simulink model "EvPowertrainController4EM"  (R2024b)
settings: configuration reference "VehicleFixed10ms" (kept outside this file)
model workspace (MAT data in the model file):
  CtrlVcuAccelPdlBpts = [0 0.8 1]
  CtrlVcuBattPnlty = 10000000
  CtrlVcuBattSOCBpts = [0 20 60 80 100]
  CtrlVcuCnstrntPnltyFctr = 10000000
  CtrlVcuEMPnlty = 100
  CtrlVcuEMTrqSplitGrid = 200
  CtrlVcuFallRate = -500
  CtrlVcuMaxAccelG = 1
  CtrlVcuMaxDecelG = -1.5
  CtrlVcuPwrDeltaPnlty = 50
  CtrlVcuPwrRatePnlty = [25 25 100]
  CtrlVcuRiseRate = 500
  CtrlVcuRoadMuEst = 0.8
  CtrlVcuSftyFctr = 0.9
  CtrlVcuTracPwrErrPnlty = 25
  CtrlVcuTrqVecBrkThresh = 0.01
  CtrlVcuTrqVecIGain = 0
  CtrlVcuTrqVecMinTrq = 25
  CtrlVcuTrqVecPGain = -2000
  CtrlVcuTrqVecSteerThresh = 0.349065850399
  CtrlVcuTrqVecVelThresh = 2.5
  N_P0 = 3
undefined symbols (not defined in the file): CtrlBcuTrlrBrkGain, CtrlVcuEvChrgLmtBpt, CtrlVcuEvRegenBrkCutOff, CtrlVcuEvRegenBrkSpdBpt, CtrlVcuEvSocBpt, eff, EnvGrvty, PlntBrkActrBoreFrnt, PlntBrkFrntBias, PlntBrkKinFricCffFrnt, PlntBrkNumPadsFrnt, PlntBrkPadMeanRadiusFrnt, PlntBrkPrsFctr, PlntBrkRearBias, PlntDiffrntl2Eff, PlntDiffrntl2Ratio, PlntDiffrntlEff, PlntDiffrntlRatio, PlntEM1EffTbl, PlntEM1Spd, PlntEM1SpdEff, PlntEM1Trq, PlntEM1TrqEff, PlntEM2EffTbl, PlntEM2Spd, PlntEM2SpdEff, PlntEM2Trq, PlntEM2TrqEff, PlntEM3EffTbl, PlntEM3Spd, PlntEM3SpdEff, PlntEM3Trq, PlntEM3TrqEff, PlntEMWhlGearEffFL, PlntEMWhlGearEffRL, PlntEMWhlGearRatioFL, PlntEMWhlGearRatioRL, PlntTransEffSpdBpt, PlntTransEffTbl, PlntTransEffTempBpt, PlntTransEffTrqBpt, PlntTransGearNumVect, PlntTransGearRatioVect, PlntVehCGHgtAxl, PlntVehDstCGFrntAxl, PlntVehDstCGRearAxl, PlntVehMass, PlntWhlLdRadiusFrnt, PlntWhlLdRadiusRear
libraries: simulink x25, autolibutils x2, slpidlib x2
(part 6 of 7)

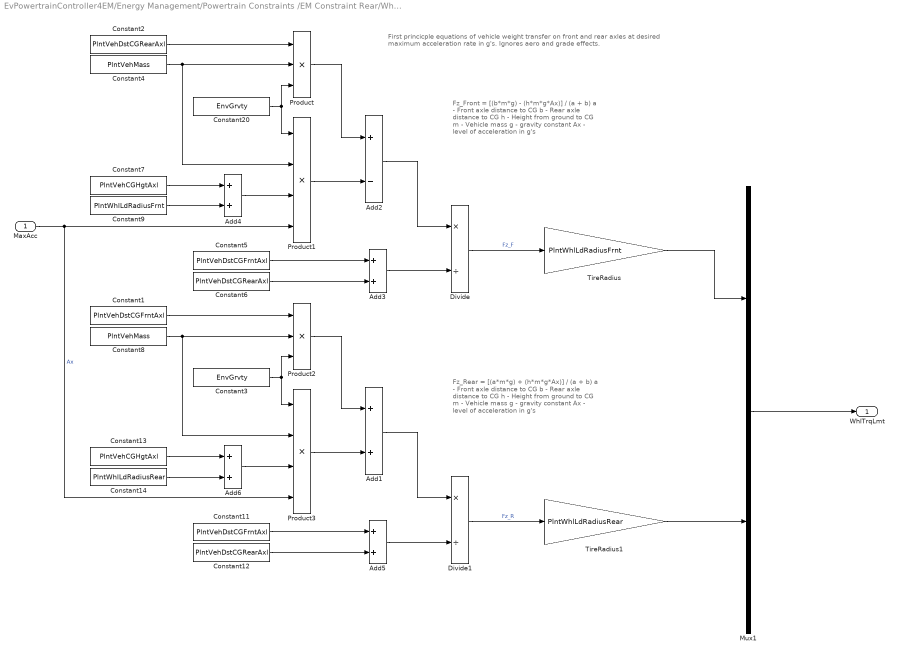
== system EvPowertrainController4EM/Energy Management/Powertrain Constraints /EM Constraint Rear/Wheel Torque Saturation for Max g Rates/Wheel Torque Limit at Max g Rates/Wheel Torque at Max Acceleration Rate ==
  note: Fz_Rear = [(a*m*g) + (h*m*g*Ax)] / (a + b)
      |
      | a - Front axle distance to CG
      | b - Rear axle distance to CG
      | h - Height from ground to CG
      | m - Vehicle mass
      | g - gravity constant
      | Ax - level of acceleration in g's
  note: Fz_Front = [(b*m*g) - (h*m*g*Ax)] / (a + b)
      |
      | a - Front axle distance to CG
      | b - Rear axle distance to CG
      | h - Height from ground to CG
      | m - Vehicle mass
      | g - gravity constant
      | Ax - level of acceleration in g's
  note: First princicple equations of vehicle weight transfer on front
      | and rear axles at desired maximum acceleration rate in g's.
      | Ignores aero and grade effects.
  MaxAcc : Inport
  Add{1,3..6} (5 alike) : Sum
  Add2 : Sum  Inputs=+-
  Constant1 : Constant  Value=PlntVehDstCGFrntAxl  SampleTime=-1
  Constant11 : Constant  Value=PlntVehDstCGFrntAxl  SampleTime=-1
  Constant12 : Constant  Value=PlntVehDstCGRearAxl  SampleTime=-1
  Constant13 : Constant  Value=PlntVehCGHgtAxl  SampleTime=-1
  Constant14 : Constant  Value=PlntWhlLdRadiusRear  SampleTime=-1
  Constant2 : Constant  Value=PlntVehDstCGRearAxl  SampleTime=-1
  Constant20 : Constant  Value=EnvGrvty  SampleTime=-1
  Constant3 : Constant  Value=EnvGrvty  SampleTime=-1
  Constant4 : Constant  Value=PlntVehMass  SampleTime=-1
  Constant5 : Constant  Value=PlntVehDstCGFrntAxl  SampleTime=-1
  Constant6 : Constant  Value=PlntVehDstCGRearAxl  SampleTime=-1
  Constant7 : Constant  Value=PlntVehCGHgtAxl  SampleTime=-1
  Constant8 : Constant  Value=PlntVehMass  SampleTime=-1
  Constant9 : Constant  Value=PlntWhlLdRadiusFrnt  SampleTime=-1
  Divide : Product  Inputs=*/
  Divide1 : Product  Inputs=*/
  Mux1 : Mux  Inputs=2
  Product : Product  Inputs=3
  Product1 : Product  Inputs=4
  Product2 : Product  Inputs=3
  Product3 : Product  Inputs=4
  TireRadius : Gain  Gain=PlntWhlLdRadiusFrnt
  TireRadius1 : Gain  Gain=PlntWhlLdRadiusRear
  WhlTrqLmt : Outport  VectorParamsAs1DForOutWhenUnconnected=off
  wires:
  Divide1/1 -> TireRadius1/1  "Fz_R"
  Product3/1 -> Add1/2
  Product2/1 -> Add1/1
  Constant11/1 -> Add5/1
  Constant8/1 -> Product3/2, Product2/2
  Add5/1 -> Divide1/2
  Add6/1 -> Product3/3
  Constant12/1 -> Add5/2
  Constant1/1 -> Product2/1
  Constant13/1 -> Add6/1
  Constant14/1 -> Add6/2
  Add1/1 -> Divide1/1
  Constant3/1 -> Product3/1, Product2/3
  Constant20/1 -> Product/3, Product1/1
  Mux1/1 -> WhlTrqLmt/1
  Add2/1 -> Divide/1
  Constant9/1 -> Add4/2
  Constant7/1 -> Add4/1
  Constant2/1 -> Product/1
  Constant6/1 -> Add3/2
  Divide/1 -> TireRadius/1  "Fz_F"
  Add4/1 -> Product1/3
  Add3/1 -> Divide/2
  MaxAcc/1 -> Product1/4, Product3/4  "Ax"
  Constant4/1 -> Product/2, Product1/2
  Constant5/1 -> Add3/1
  Product/1 -> Add2/1
  Product1/1 -> Add2/2
  TireRadius/1 -> Mux1/1
  TireRadius1/1 -> Mux1/2

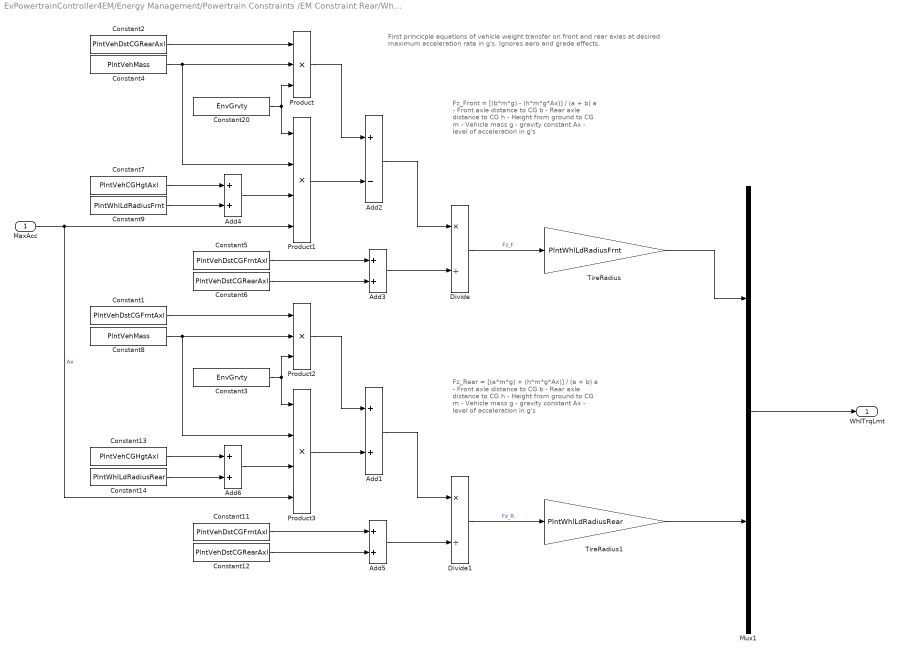
== system EvPowertrainController4EM/Energy Management/Powertrain Constraints /EM Constraint Rear/Wheel Torque Saturation for Max g Rates/Wheel Torque Limit at Max g Rates/Wheel Torque at Max Deceleration Rate ==
  note: First princicple equations of vehicle weight transfer on front
      | and rear axles at desired maximum acceleration rate in g's.
      | Ignores aero and grade effects.
  note: Fz_Front = [(b*m*g) - (h*m*g*Ax)] / (a + b)
      |
      | a - Front axle distance to CG
      | b - Rear axle distance to CG
      | h - Height from ground to CG
      | m - Vehicle mass
      | g - gravity constant
      | Ax - level of acceleration in g's
  note: Fz_Rear = [(a*m*g) + (h*m*g*Ax)] / (a + b)
      |
      | a - Front axle distance to CG
      | b - Rear axle distance to CG
      | h - Height from ground to CG
      | m - Vehicle mass
      | g - gravity constant
      | Ax - level of acceleration in g's
  MaxAcc : Inport
  Add{1,3..6} (5 alike) : Sum
  Add2 : Sum  Inputs=+-
  Constant1 : Constant  Value=PlntVehDstCGFrntAxl  SampleTime=-1
  Constant11 : Constant  Value=PlntVehDstCGFrntAxl  SampleTime=-1
  Constant12 : Constant  Value=PlntVehDstCGRearAxl  SampleTime=-1
  Constant13 : Constant  Value=PlntVehCGHgtAxl  SampleTime=-1
  Constant14 : Constant  Value=PlntWhlLdRadiusRear  SampleTime=-1
  Constant2 : Constant  Value=PlntVehDstCGRearAxl  SampleTime=-1
  Constant20 : Constant  Value=EnvGrvty  SampleTime=-1
  Constant3 : Constant  Value=EnvGrvty  SampleTime=-1
  Constant4 : Constant  Value=PlntVehMass  SampleTime=-1
  Constant5 : Constant  Value=PlntVehDstCGFrntAxl  SampleTime=-1
  Constant6 : Constant  Value=PlntVehDstCGRearAxl  SampleTime=-1
  Constant7 : Constant  Value=PlntVehCGHgtAxl  SampleTime=-1
  Constant8 : Constant  Value=PlntVehMass  SampleTime=-1
  Constant9 : Constant  Value=PlntWhlLdRadiusFrnt  SampleTime=-1
  Divide : Product  Inputs=*/
  Divide1 : Product  Inputs=*/
  Mux1 : Mux  Inputs=2
  Product : Product  Inputs=3
  Product1 : Product  Inputs=4
  Product2 : Product  Inputs=3
  Product3 : Product  Inputs=4
  TireRadius : Gain  Gain=PlntWhlLdRadiusFrnt
  TireRadius1 : Gain  Gain=PlntWhlLdRadiusRear
  WhlTrqLmt : Outport  VectorParamsAs1DForOutWhenUnconnected=off
  wires:
  TireRadius1/1 -> Mux1/2
  TireRadius/1 -> Mux1/1
  Product1/1 -> Add2/2
  Product/1 -> Add2/1
  Constant5/1 -> Add3/1
  Constant4/1 -> Product1/2, Product/2
  MaxAcc/1 -> Product3/4, Product1/4  "Ax"
  Add3/1 -> Divide/2
  Add4/1 -> Product1/3
  Divide/1 -> TireRadius/1  "Fz_F"
  Constant6/1 -> Add3/2
  Constant2/1 -> Product/1
  Constant7/1 -> Add4/1
  Constant9/1 -> Add4/2
  Add2/1 -> Divide/1
  Mux1/1 -> WhlTrqLmt/1
  Constant20/1 -> Product1/1, Product/3
  Constant3/1 -> Product2/3, Product3/1
  Add1/1 -> Divide1/1
  Constant14/1 -> Add6/2
  Constant13/1 -> Add6/1
  Constant1/1 -> Product2/1
  Constant12/1 -> Add5/2
  Add6/1 -> Product3/3
  Add5/1 -> Divide1/2
  Constant8/1 -> Product2/2, Product3/2
  Constant11/1 -> Add5/1
  Product2/1 -> Add1/1
  Product3/1 -> Add1/2
  Divide1/1 -> TireRadius1/1  "Fz_R"

== system EvPowertrainController4EM/Energy Management/Powertrain Constraints /EM Constraint Front/Tabular Power Loss Data/2EM or 3EM Dual Rear/WhlTrq2EMTrq/Diff Eta ==
  note: Pwr >= 0, v = 1
      | Pwr < 0, v= -1
  SpdIn : Inport
  TrqIn : Inport  Port=2
  Constant : Constant  Value=PlntDiffrntl2Eff
  Constant1 : Constant  SampleTime=-1
  Constant2 : Constant  Value=-1  SampleTime=-1
  Math Function1 : Math  Operator=pow  SignedPower=on  OutputSignalType=real
  Product1 : Product
  Switch2 : Switch  SaturateOnIntegerOverflow=off  InputSameDT=off
  eta : Outport  VectorParamsAs1DForOutWhenUnconnected=off
  wires:
  SpdIn/1 -> Product1/2
  Constant/1 -> Math Function1/1
  Constant2/1 -> Switch2/3
  Constant1/1 -> Switch2/1
  Product1/1 -> Switch2/2
  Switch2/1 -> Math Function1/2
  Math Function1/1 -> eta/1
  TrqIn/1 -> Product1/1

== system EvPowertrainController4EM/Energy Management/Powertrain Constraints /EM Constraint Front/Tabular Power Loss Data/3EM Dual Front or 4EM/WhlTrq2EMTrq/Gear Eta ==
  note: Pwr >= 0, v = 1
      | Pwr < 0, v= -1
  SpdIn : Inport
  TrqIn : Inport  Port=2
  Constant : Constant  Value=PlntEMWhlGearEffRL
  Constant1 : Constant  SampleTime=-1
  Constant2 : Constant  Value=-1  SampleTime=-1
  Math Function1 : Math  Operator=pow  SignedPower=on  OutputSignalType=real
  Product1 : Product
  Switch2 : Switch  SaturateOnIntegerOverflow=off  InputSameDT=off
  eta : Outport  VectorParamsAs1DForOutWhenUnconnected=off
  wires:
  TrqIn/1 -> Product1/1
  Math Function1/1 -> eta/1
  Switch2/1 -> Math Function1/2
  Product1/1 -> Switch2/2
  Constant1/1 -> Switch2/1
  Constant2/1 -> Switch2/3
  Constant/1 -> Math Function1/1
  SpdIn/1 -> Product1/2

== system EvPowertrainController4EM/Energy Management/Powertrain Constraints /EM Constraint Rear/Tabular Power Loss Data/2EM/WhlTrq2EMTrq/Diff Eta ==
  note: Pwr >= 0, v = 1
      | Pwr < 0, v= -1
  SpdIn : Inport
  TrqIn : Inport  Port=2
  Constant : Constant  Value=PlntDiffrntl2Eff
  Constant1 : Constant  SampleTime=-1
  Constant2 : Constant  Value=-1  SampleTime=-1
  Math Function1 : Math  Operator=pow  SignedPower=on  OutputSignalType=real
  Product1 : Product
  Switch2 : Switch  SaturateOnIntegerOverflow=off  InputSameDT=off
  eta : Outport  VectorParamsAs1DForOutWhenUnconnected=off
  wires:
  SpdIn/1 -> Product1/2
  Constant/1 -> Math Function1/1
  Constant2/1 -> Switch2/3
  Constant1/1 -> Switch2/1
  Product1/1 -> Switch2/2
  Switch2/1 -> Math Function1/2
  Math Function1/1 -> eta/1
  TrqIn/1 -> Product1/1

== system EvPowertrainController4EM/Energy Management/Powertrain Constraints /EM Constraint Rear/Tabular Power Loss Data/3EM Dual Front/WhlTrq2EMTrq/Diff Eta ==
  note: Pwr >= 0, v = 1
      | Pwr < 0, v= -1
  SpdIn : Inport
  TrqIn : Inport  Port=2
  Constant : Constant  Value=PlntDiffrntl2Eff
  Constant1 : Constant  SampleTime=-1
  Constant2 : Constant  Value=-1  SampleTime=-1
  Math Function1 : Math  Operator=pow  SignedPower=on  OutputSignalType=real
  Product1 : Product
  Switch2 : Switch  SaturateOnIntegerOverflow=off  InputSameDT=off
  eta : Outport  VectorParamsAs1DForOutWhenUnconnected=off
  wires:
  TrqIn/1 -> Product1/1
  Math Function1/1 -> eta/1
  Switch2/1 -> Math Function1/2
  Product1/1 -> Switch2/2
  Constant1/1 -> Switch2/1
  Constant2/1 -> Switch2/3
  Constant/1 -> Math Function1/1
  SpdIn/1 -> Product1/2

== system EvPowertrainController4EM/Energy Management/Powertrain Constraints /EM Constraint Rear/Tabular Power Loss Data/3EM Dual Rear or 4EM/WhlTrq2EMTrq/Gear Eta ==
  note: Pwr >= 0, v = 1
      | Pwr < 0, v= -1
  SpdIn : Inport
  TrqIn : Inport  Port=2
  Constant : Constant  Value=PlntEMWhlGearEffRL
  Constant1 : Constant  SampleTime=-1
  Constant2 : Constant  Value=-1  SampleTime=-1
  Math Function1 : Math  Operator=pow  SignedPower=on  OutputSignalType=real
  Product1 : Product
  Switch2 : Switch  SaturateOnIntegerOverflow=off  InputSameDT=off
  eta : Outport  VectorParamsAs1DForOutWhenUnconnected=off
  wires:
  TrqIn/1 -> Product1/1
  Math Function1/1 -> eta/1
  Switch2/1 -> Math Function1/2
  Product1/1 -> Switch2/2
  Constant1/1 -> Switch2/1
  Constant2/1 -> Switch2/3
  Constant/1 -> Math Function1/1
  SpdIn/1 -> Product1/2

== matlab function EvPowertrainController4EM/Torque Vectoring/3EM/Torque Vectoring Split Function ==
  data: MaxTrq input; TrqLeftOut output; TrqLeft input; TrqRght input; TrqRghtOut output; TrqVec input; Enbl input; BrkThresh input; MinTrq input
function [TrqLeftOut, TrqRghtOut] = fcn(MaxTrq, TrqLeft, TrqRght, TrqVec, Enbl, BrkThresh, MinTrq)
% Enbl:= flag to turn on TV, true if steering wheel is turned and non-zero vehicle speed
% BrkThresh:= flag to turn on TV, true if not braking
TrqLmt = min(MaxTrq-abs(TrqLeft),MaxTrq-abs(TrqRght));
DeltaTrq = min(MinTrq, min(TrqLmt,abs(TrqVec)))*sign(TrqVec)*Enbl;% limit difference in torque between tires to +/-MinTrq and to max/min motor torque
if BrkThresh > 0 % Not braking. Use Torque vectoring
    TrqLeftOut = (TrqLeft+DeltaTrq);
    TrqRghtOut = (TrqRght-DeltaTrq);
else % ignore TV
    TrqLeftOut = TrqLeft;
    TrqRghtOut = TrqRght;
end

== matlab function EvPowertrainController4EM/Torque Vectoring/4EM/Torque Vectoring Split Function Rear ==
  data: MaxTrq input; TrqLeftOut output; TrqLeft input; TrqRght input; TrqRghtOut output; TrqVec input; Enbl input; BrkThresh input; MinTrq input
function [TrqLeftOut, TrqRghtOut] = fcn(MaxTrq, TrqLeft, TrqRght, TrqVec, Enbl, BrkThresh, MinTrq)
% Enbl:= flag to turn on TV, true if steering wheel is turned and non-zero vehicle speed
% BrkThresh:= flag to turn on TV, true if not braking
TrqLmt = min(MaxTrq-abs(TrqLeft),MaxTrq-abs(TrqRght));
DeltaTrq = min(MinTrq, min(TrqLmt,abs(TrqVec)))*sign(TrqVec)*Enbl;% limit difference in torque between tires to +/-MinTrq and to max/min motor torque
if BrkThresh > 0 % Not braking. Use Torque vectoring
    TrqLeftOut = (TrqLeft+DeltaTrq);
    TrqRghtOut = (TrqRght-DeltaTrq);
else % ignore TV
    TrqLeftOut = TrqLeft;
    TrqRghtOut = TrqRght;
end

== matlab function EvPowertrainController4EM/Torque Vectoring/LTV_MPC/LTV_MPCFcn ==
  data: Acc input; delta_Frnt input; TV_enableflag input; xk input; PrevEMTrqCmdFinals input; EMTrqCmds input; Vx input; EMTrqMaxFrnt input; EMTrqMaxRear input; xi_in input; EMTrqCmdFinal output; xhat_kp1 output; fval output; exitflag output; allCosts output; compTime output; stepSize output; iterations output; funcCount output; betaMax output; r_ref output; xi_out output
function [EMTrqCmdFinal, xhat_kp1, fval, exitflag, allCosts, compTime, stepSize, iterations, funcCount, betaMax, r_ref, xi_out] ...
    = LTV_MPC(Acc, delta_Frnt, TV_enableflag, xk, PrevEMTrqCmdFinals, EMTrqCmds, Vx, EMTrqMaxFrnt, EMTrqMaxRear, xi_in)

%% MPC Tuning Parameters
Np = 10;    % prediction horizon [interval]
Nc = 3;     % control horizon [interval] 

% % -----------------------------------------------------------------

Q_y = 100;      % Yaw rate tracking weight
Q_T = eye(4);  % Torque increment (slew rate) weight

% % -----------------------------------------------------------------

% % % Allowed Maximum MPC computation Iterations
Iter_max = 300;

%% Defining fixed parameter structure
nx = 2; % number of states
nu = 2; % number of controls

% % System parameters
m  = 1623;          % [kg]           % vehicle mass
Iz = 2066;          % [kg m^2]       % yaw moment of inertia
lf = 1.09;          % [m]            % distance from c.o.g. to front axle
lr = 1.7;           % [m]            % distance from c.o.g. to rear axle
lw = 1.575;         % [m]            % track width
rw = 0.309;         % [m]            % wheel radius
h  = 0.609;         % [m]            % distance from c.o.g. to ground
g  = 9.81;          % [m/s^2]        % gravitational acceleration

mu_x = 0.8*0.9;     % assumed tire-road friction coefficient

% % Tires' magic formula coefficients
D = 1.0;    % []            % peak factor scale
C = 1.1;    % []            % shape factor
E = 1.2;    % []            % curvature factor

EMWhlGearRatio = 0.98*4.1; % (wheel torque = efficiency * final gear * motor torque)

EMTrqIncMax = 500*0.01.*ones(4,1); % sampling time = 0.01 [s];

EMFrntTrq = EMTrqCmds(1) + EMTrqCmds(2); % front axle (motor) torque
EMRearTrq = EMTrqCmds(3) + EMTrqCmds(4); % rear  axle (motor) torque

%% System bounds
% % Maximum side slip angle
Car = 2.4E4; % (estimated) rear cornering stiffness
betaMax = abs(mu_x*g*(lr/Vx^2 + m*lf/(Car*(lf+lr))));

%% Yaw rate reference
% Neutral steer
r_ref = Vx*delta_Frnt/(lf+lr);

% Maximum yaw rate reference
r_ref_max = abs(0.85* mu_x*g/(Vx+1e-6)); 

% Saturated reference
if abs(r_ref) > r_ref_max
    r_ref = r_ref_max*sign(delta_Frnt);
end

%% Provide an initial guess by shifting the previous solution 1 step (Warm Start)
% Calculate indices for clarity
% Controls
control_end = nu*Nc;
% States
state_end   = control_end + nx*Np;

% Construct the warm start vector by shifting previous solution
xi_0 = [xi_in(nu+1 : control_end);              % shifted controls (skip first control)
        xi_in(control_end-nu+1 : control_end);  % repeat last control
        xi_in(control_end+nx+1 : state_end);    % shifted states (skip first state)
        xi_in(state_end-nx+1 : state_end)];      % repeat last state

%% Fixed parameter structure
params = struct('m',m,'Iz',Iz,'lf',lf,'lr',lr,'lw',lw,'rw',rw,'h',h,'g',g, ...
    'D', D, 'C', C, 'E', E, 'mu_x',mu_x, 'EMWhlGearRatio',EMWhlGearRatio);

%% MPC Call

% % Solver settings

% % quadprog settings
% opts = optimoptions("quadprog","Algorithm","active-set","MaxIterations",Iter_max); 

% % mpcActiveSetSolver settings
opts2 = mpcActiveSetOptions('double');
opts2.MaxIterations = Iter_max;
opts2.ConstraintTolerance = 1e-5;

% % default outputs

EMTrqCmdFinal = EMTrqCmds;

xi_out      = [kron(ones(Nc,1), [0;0]); % control
               kron(ones(Np,1), xk)];      % states

xhat_kp1    = xk;
allCosts    = 0;
exitflag    = int32(0); % 0 for quadprog
fval        = 0;
compTime    = 0;
stepSize    = 0;
iterations  = 0;
funcCount   = 0;

maxLinearizationUpdates = 3;

% % % If Torque Vectoring is enable, use MPC to re-compute outputs
if TV_enableflag > 0

    Ts = 0.01; % discretization time

    A_list = cell(Np,1); 
    B_list = cell(Np,1); 
    K_list = cell(Np,1);

    xi = xi_0;

    timeStart = tic;
    for iter = 1:maxLinearizationUpdates
        % Step 1: get x_star, u_star from xi
        x_seq0 = reshape(xi(nu*Nc+1:end), nx, Np);
        u_seq0 = reshape(xi(1:nu*Nc), nu, Nc);
    
        % Step 2: update dynamics
        for k = 1:Np
            if k == 1
                x_star_k = xk;
            else
                x_star_k = x_seq0(:,k);
            end
            u_star_k = u_seq0(:,min(k,Nc));
            At = A_(x_star_k, Vx, delta_Frnt, Acc, mu_x);
            Bt = B_(delta_Frnt);
            fxu = MPC_getVehicleDynamics(x_star_k, u_star_k, EMFrntTrq, Vx, delta_Frnt, Acc, params);
            A_list{k} = eye(nx) + Ts * At;
            B_list{k} = Ts * Bt;
            K_list{k} = Ts * (fxu - At*x_star_k - Bt*u_star_k);
        end
    
        % Step 3: update constraints & cost
        % Build cost matrix
        [H, f] = buildCostMatrices(EMFrntTrq, EMRearTrq, ...
                                            PrevEMTrqCmdFinals, r_ref, Q_y, Q_T, Np, Nc, nx, nu);
    
        H = 0.5*(H + H.'); % symmetrize the Hessian matrix
        H = 2.*H + 1e-6 * eye(size(H)); % max(abs(diag(H))) Regularize the Hessian matrix
    
        % Build equality constraint matrix
        [Aeq, beq] = buildEqualityConstraints(xk, A_list, B_list, K_list, Np, Nc, nx, nu);
    
        % Build inequality constraint matrix
        [Aineq, bineq] = buildInequalityConstraints(PrevEMTrqCmdFinals, EMFrntTrq, EMRearTrq, ...
                                        EMTrqMaxFrnt, EMTrqMaxRear, EMTrqIncMax, delta_Frnt, Vx, betaMax, Np, Nc, nx, nu);
    
        % Step 4: Solve OCP
    
        % [xi_new, fval, exitflag, ~] = quadprog(H,f,Aineq,bineq,Aeq,beq,[], [], xi, opts);
    
        iA0 = false(size(bineq));
        [xi_new, exitflag] = mpcActiveSetSolver(H, f, Aineq, bineq, Aeq, beq, iA0, opts2);
    
        % Step 5: check convergence
        if norm(xi_new - xi, Inf) < 1e-3
            break;
        end
        
        xi = xi_new;
    end
    
    compTime = toc(timeStart);
    
    xi_out = xi_new;

    % % Extract optimal controls
    EMTrqCmdFinal = getEMTrqs(EMFrntTrq, EMRearTrq, xi_out(1:nu));

    % % Obtain optimal (predicted) next state
    xhat_kp1 = A_list{1}*xk + B_list{1}*xi_out(1:nu) + K_list{1};

end

% % % --------------------- end of main program ----------------------

% % % ----------------------- begin of costs -----------------------

%% Cost Function

function [H, f] = buildCostMatrices(EMFrntTrq, EMRearTrq, ...
                                        PrevEMTrqCmdFinals, r_ref, Q_y, Q_T, Np, Nc, nx, nu)
    % Q_T: 4x4 matrix weighting torque increment per wheel

    Nvar = nu*Nc + nx*Np;
    H = zeros(Nvar, Nvar);
    f = zeros(Nvar, 1);

    % % 1. Yaw rate tracking cost
    for k = 1:Np
        yaw_idx = nu*Nc + (k-1)*nx + 2; % index of yaw rate
        H(yaw_idx, yaw_idx) = Q_y;
        f(yaw_idx) = - 2 * Q_y * r_ref;
    end

    % % 2. Torque increment cost in terms of actual wheel torques
    M = [-0.5  0;
          0.5  0;
          0   -0.5;
          0    0.5]; % 4x2 matrix

    W = M.' * Q_T * M; % Effective weight in uk space

    for k = 1:Nc
        uk_idx = (k-1)*nu + (1:nu);

        if k == 1
            % T_0 = PrevEMTrqCmdFinals (fixed)
            T_prev = PrevEMTrqCmdFinals;

            % C_1 = 0.5*[F; F; R; R]
            C1 = 0.5 * [EMFrntTrq; EMFrntTrq; EMRearTrq; EMRearTrq];

            offset = C1 - T_prev;

            H(uk_idx, uk_idx) = H(uk_idx, uk_idx) + W;
            f(uk_idx) = f(uk_idx) + 2 * M' * Q_T * offset;

        else
            ukm1_idx = (k-2)*nu + (1:nu);
            H(uk_idx, uk_idx)     = H(uk_idx, uk_idx)     + W;
            H(ukm1_idx, ukm1_idx) = H(ukm1_idx, ukm1_idx) + W;
            H(uk_idx, ukm1_idx)   = H(uk_idx, ukm1_idx)   - W;
            H(ukm1_idx, uk_idx)   = H(ukm1_idx, uk_idx)   - W;
        end
    end
% end

% % % --------------------- end of costs ----------------------


% % % --------------------- begin of constraints -----------------------

%% Equality Constraint Function

function [Aeq, beq] = buildEqualityConstraints(xk, A_list, B_list, K_list, Np, Nc, nx, nu)
    % Total number of variables
    Nvar = nu*Nc + nx*Np;

    % Preallocate
    Aeq = zeros(nx*Np, Nvar);
    beq = zeros(nx*Np, 1);

    for k = 1:Np
        row_idx = (k-1)*nx + (1:nx); % rows for stage k

        % Extract system matrices
        Ak = A_list{k};
        Bk = B_list{k};
        Kk = K_list{k};

        if k == 1
            % First dynamics constraint: x1 = A0*xk + B0*u0 + K0
            u_idx = (0)*nu + (1:nu);
            x_idx = nu*Nc + (k-1)*nx + (1:nx);

            Aeq(row_idx, u_idx) = -Bk;
            Aeq(row_idx, x_idx) = eye(nx);
            beq(row_idx) = Kk + Ak * xk;

        else
            % k ≥ 2: x_k = A_{k-1} * x_{k-1} + B_{k-1} * u_{k-1} + K_{k-1}
            u_idx = min(k-1,Nc-1)*nu + (1:nu);
            x_prev_idx = nu*Nc + (k-2)*nx + (1:nx);
            x_curr_idx = nu*Nc + (k-1)*nx + (1:nx);

            Aeq(row_idx, u_idx)       = -Bk;
            Aeq(row_idx, x_prev_idx)  = -Ak;
            Aeq(row_idx, x_curr_idx)  = eye(nx);
            beq(row_idx)              = Kk;
        end
    end
% end

%% Inequality Constraint Function
function [Aineq, bineq] = buildInequalityConstraints(PrevEMTrqCmdFinals, EMFrntTrq, EMRearTrq, ...
                                    EMTrqMaxFrnt, EMTrqMaxRear, EMTrqIncMax, delta_Frnt, Vx, betaMax, Np, Nc, nx, nu)

    % Dimensions
    Nvar = nu*Nc + nx*Np;

    % % 1. Individual torque increment constraint: |T_k - T_{k-1}| <= ΔT_max
    A_dT = zeros(0,Nvar);
    b_dT = zeros(0,1);

    % Mapping from control to individual torque: T = C_k + M*u_k
    M = [-0.5  0;
          0.5  0;
          0   -0.5;
          0    0.5];  % size 4x2

    for k = 1:Nc
        idx = (k-1)*nu + (1:nu);

        % Affine offsets
        Ck = 0.5 * [EMFrntTrq; EMFrntTrq; EMRearTrq; EMRearTrq];

        if k == 1
            % First step: T_0 = PrevEMTrqCmdFinals
            dC = Ck - PrevEMTrqCmdFinals;
            E = zeros(4, Nvar);
            E(:, idx) = M;

            A_dT = [A_dT;
                     E;
                    -E];
            b_dT = [b_dT;
                    EMTrqIncMax - dC;
                    EMTrqIncMax + dC];

        else
            % Use difference u_k - u_{k-1}
            idx_prev = (k-2)*nu + (1:nu);
            dC = [0; 0; 0; 0];  % if EMFrntTrq/R are constant

            E = zeros(4, Nvar);
            E(:, idx) =  M;
            E(:, idx_prev) = -M;

            A_dT = [A_dT;
                     E;
                    -E];
            b_dT = [b_dT;
                    EMTrqIncMax - dC;
                    EMTrqIncMax + dC];
        end
    end

    % % 2. EMTrq magnitude constraint (corrected affine form)
    A_trq = zeros(0, Nvar);
    b_trq = zeros(0, 1);

    M = [-0.5  0;
          0.5  0;
          0   -0.5;
          0    0.5];  % 4x2

    EMTrqsMax = [EMTrqMaxFrnt; EMTrqMaxFrnt; EMTrqMaxRear; EMTrqMaxRear];

    for k = 1:Nc
        idx = (k-1)*nu + (1:nu);

        % Constant part from fixed front/rear torques
        c_k = 0.5 * [EMFrntTrq; EMFrntTrq; EMRearTrq; EMRearTrq];

        E = zeros(4, Nvar);
        E(:, idx) = M;

        A_trq = [A_trq;
                 E;      % M * u_k <= EMTrqsMax - c_k
                -E];     % -M * u_k <= EMTrqsMax + c_k

        b_trq = [b_trq;
                 EMTrqsMax - c_k;
                 EMTrqsMax + c_k];
    end

    % % 3. Vectoring encouragement: -uk(1)*delta <= 0, -uk(2)*delta <= 0
    % This encourages uk(i) * delta >= 0

    A_vec = zeros(0, Nvar);%[];
    b_vec = zeros(0, 1);%[];

    for k = 1:Nc
        idx = (k-1)*nu + (1:nu);
        E = zeros(2, Nvar);
        E(1, idx(1)) = -delta_Frnt;
        E(2, idx(2)) = -delta_Frnt;

        A_vec = [A_vec; E];
        b_vec = [b_vec; zeros(2,1)];
    end
    
    % % 4. Vectoring torque bound: |u_k| <= 2 * [EMTrqMaxFrnt; EMTrqMaxRear]
    A_vecMag = zeros(0, Nvar);
    b_vecMag = zeros(0, 1);

    u_bound = [2*EMTrqMaxFrnt; 2*EMTrqMaxRear];

    for k = 1:Nc
        idx = (k-1)*nu + (1:nu);
        E = zeros(nu, Nvar);
        E(:, idx) = eye(nu);

        A_vecMag = [A_vecMag;
                    E;
                   -E];
        b_vecMag = [b_vecMag;
                    u_bound;
                    u_bound];
    end

    % % 5. Body slip angle constraint: |Vy_k| <= Vx * tan(beta_max)
    A_beta = zeros(0, Nvar);
    b_beta = zeros(0, 1);
    
    Vy_bound = Vx * tan(betaMax);
    
    for k = 1:Np
        xk_idx = nu*Nc + (k-1)*nx + 1; % Vy index
        
        E = zeros(1, Nvar);
        E(1, xk_idx) = 1;
        A_beta = [A_beta; 
                  E;
                 -E];
        b_beta = [b_beta; 
                  Vy_bound;
                  Vy_bound];
    end
    
    % % % 6. yaw rate constraint: |r_k| <= r_max
    % A_r = zeros(0, Nvar);
    % b_r = zeros(0, 1);
    % 
    % r_max = 1;
    % 
    % for k = 1:Np
    %     xk_idx = nu*Nc + (k-1)*nx + 2; % r index
    % 
    %     E = zeros(1, Nvar);
    %     E(1, xk_idx) = 1;
    %     A_r = [A_r; 
    %            E;
    %           -E];
    %     b_r = [b_r; 
    %            r_max;
    %            r_max];
    % end

    % % Combine all inequality constraints
    Aineq = [A_dT; A_trq; A_vec; A_vecMag; A_beta];% A_r];
    bineq = [b_dT; b_trq; b_vec; b_vecMag; b_beta];% b_r];

% end

% % % --------------------- end of constraints ----------------------

% % % --------------------- begin of dynamics -----------------------

function xk_dot = MPC_getVehicleDynamics(xk, uk, EMFrntTrq, Vx, delta_Frnt, Acc, params)

% % System parameters
m = params.m;           % [kg]           % vehicle mass
Iz = params.Iz;         % [kg m^2]       % yaw moment of inertia
lf = params.lf;         % [m]            % distance from c.o.g. to front axle
lr = params.lr;         % [m]            % distance from c.o.g. to rear axle
lw = params.lw;         % [m]            % track width
rw = params.rw;         % [m]            % wheel radius

% Get lateral forces
[Fy, ~] = getForces(xk, Vx, delta_Frnt, Acc, params);
Fy_FL = Fy(1); Fy_FR = Fy(2); Fy_RL = Fy(3); Fy_RR = Fy(4);

% % Continuous-time dynamics
Vy_dot = ( (EMFrntTrq*params.EMWhlGearRatio/rw)*sin(delta_Frnt) + (Fy_FL+Fy_FR)*cos(delta_Frnt) + Fy_RL + Fy_RR)/m - Vx*xk(2);

r_dot = ( ( (EMFrntTrq*params.EMWhlGearRatio/rw)*sin(delta_Frnt) + (Fy_FL+Fy_FR)*cos(delta_Frnt) )*lf ...
            + ( (uk(1)*params.EMWhlGearRatio/rw)*cos(delta_Frnt) + (Fy_FL-Fy_FR)*sin(delta_Frnt) )*lw/2 ...
            + (uk(2)*params.EMWhlGearRatio/rw)*lw/2 - (Fy_RL+Fy_RR)*lr)/Iz;
xk_dot = [Vy_dot; r_dot];

% end

% % -----------------------------------------------------------------

function [Fy, Fz] = getForces(xk, Vx, delta_Frnt, Acc, params)
% % System parameters
m = params.m;           % [kg]           % vehicle mass
lf = params.lf;         % [m]            % distance from c.o.g. to front axle
lr = params.lr;         % [m]            % distance from c.o.g. to rear axle
lw = params.lw;         % [m]            % track width
h  = params.h;          % [m]            % distance from c.o.g. to ground
g  = params.g;          % [m/s^2]        % gravitational acceleration
mu = params.mu_x;       % []             % friction coefficient

% % Tires' magic formula coefficients
D = params.D; % []           % peak factor scale
C = params.C; % []            % shape factor
E = params.E; % []            % curvature factor

% % Compute Vertical Loads
Fz_FL = 0.5*( m*g*lr/(lf+lr) - m*Acc(1)*h/(lf+lr) - m*-Acc(2)*h*lr/(lw*(lf+lr)) );
Fz_FR = 0.5*( m*g*lr/(lf+lr) - m*Acc(1)*h/(lf+lr) + m*-Acc(2)*h*lr/(lw*(lf+lr)) );
Fz_RL = 0.5*( m*g*lf/(lf+lr) + m*Acc(1)*h/(lf+lr) - m*-Acc(2)*h*lf/(lw*(lf+lr)) );
Fz_RR = 0.5*( m*g*lf/(lf+lr) + m*Acc(1)*h/(lf+lr) + m*-Acc(2)*h*lf/(lw*(lf+lr)) );
Fz = [Fz_FL; Fz_FR; Fz_RL; Fz_RR];

% Compute wheel side slip angles
[a_FL,a_FR,a_RL,a_RR] = getTireSlipAng(xk, Vx, delta_Frnt, params);

% % Lateral forces
Fy = [ mu*D*Fz_FL*sin( C*atan( ( 4E4/(mu*D*Fz_FL)  ) *a_FL - E*( ( 4E4/(mu*D*Fz_FL)  ) *a_FL - atan( ( 4E4/(mu*D*Fz_FL)  ) *a_FL ) ) ) );
       mu*D*Fz_FR*sin( C*atan( ( 4E4/(mu*D*Fz_FR)  ) *a_FR - E*( ( 4E4/(mu*D*Fz_FR)  ) *a_FR - atan( ( 4E4/(mu*D*Fz_FR)  ) *a_FR ) ) ) );
       mu*D*Fz_RL*sin( C*atan( ( 4E4/(mu*D*Fz_RL)  ) *a_RL - E*( ( 4E4/(mu*D*Fz_RL)  ) *a_RL - atan( ( 4E4/(mu*D*Fz_RL)  ) *a_RL ) ) ) );
       mu*D*Fz_RR*sin( C*atan( ( 4E4/(mu*D*Fz_RR)  ) *a_RR - E*( ( 4E4/(mu*D*Fz_RR)  ) *a_RR - atan( ( 4E4/(mu*D*Fz_RR)  ) *a_RR ) ) ) )    ];

% end

% % -----------------------------------------------------------------

function [a_FL,a_FR,a_RL,a_RR] = getTireSlipAng(xk, Vx, delta_Frnt, params)
% % System parameters
lf = params.lf;         % [m]            % distance from c.o.g. to front axle
lr = params.lr;         % [m]            % distance from c.o.g. to rear axle
lw = params.lw;         % [m]            % track width

% a_FL = -atan2((xk(1) + xk(2)*lf),(Vx - xk(2)*lw/2)) + delta_Frnt;        % front-left
% a_FR = -atan2((xk(1) + xk(2)*lf),(Vx + xk(2)*lw/2)) + delta_Frnt;        % front-right
% a_RL = -atan2((xk(1) - xk(2)*lr),(Vx - xk(2)*lw/2));                     % rear-left
% a_RR = -atan2((xk(1) - xk(2)*lr),(Vx + xk(2)*lw/2));                     % rear-right

a_FL = -atan((xk(1) + xk(2)*lf)/(Vx - xk(2)*lw/2)) + delta_Frnt;        % front-left
a_FR = -atan((xk(1) + xk(2)*lf)/(Vx + xk(2)*lw/2)) + delta_Frnt;        % front-right
a_RL = -atan((xk(1) - xk(2)*lr)/(Vx - xk(2)*lw/2));                     % rear-left
a_RR = -atan((xk(1) - xk(2)*lr)/(Vx + xk(2)*lw/2));                     % rear-right

% end

% % -----------------------------------------------------------------

function EMTrqs = getEMTrqs(EMFrntTrq, EMRearTrq, uk)
EMTrqs = [  0.5*(EMFrntTrq - uk(1)); % EMTrq_FL
            0.5*(EMFrntTrq + uk(1)); % EMTrq_FR
            0.5*(EMRearTrq - uk(2)); % EMTrq_RL
            0.5*(EMRearTrq + uk(2))  ]; % EMTrq_RR
% end

% % % --------------------- end of dynamics ----------------------

function gradfx = A_(in1,Vx,delta,in4,mu)
%A_
%    GRADFX = A_(IN1,Vx,DELTA,IN4,MU)

%    This function was generated by the Symbolic Math Toolbox version 24.2.
%    28-Jun-2025 15:18:14

Acc1 = in4(1,:);
Acc2 = in4(2,:);
xk1 = in1(1,:);
xk2 = in1(2,:);
t2 = cos(delta);
t3 = sin(delta);
t4 = 1.0./mu;
t6 = xk2.*(1.7e+1./1.0e+1);
t8 = xk2.*(6.3e+1./8.0e+1);
t10 = xk2.*(1.09e+2./1.0e+2);
t17 = Acc1.*1.771338709677419e+2;
t18 = Acc2.*1.911921146953405e+2;
t24 = Acc2.*1.225878853046595e+2;
t5 = t4.^2;
t9 = -t8;
t11 = Vx+t8;
t14 = t10+xk1;
t15 = (t6-xk1).^2;
t21 = -t17;
t25 = -t24;
t69 = t17+t18-4.850675806451613e+3;
t70 = t17+t24+3.110139193548388e+3;
t13 = Vx+t9;
t16 = t14.^2;
t19 = 1.0./t11;
t68 = t18+t21+4.850675806451613e+3;
t71 = t17+t25+3.110139193548388e+3;
t73 = 1.0./t69;
t76 = 1.0./t70;
t20 = t19.^2;
t22 = 1.0./t13;
t26 = t19.*(1.7e+1./1.0e+1);
t28 = t19.*(1.09e+2./1.0e+2);
t30 = -t19.*(t6-xk1);
t33 = t14.*t19;
t72 = 1.0./t68;
t75 = t73.^2;
t77 = t76.^2;
t78 = 1.0./t71;
t23 = t22.^2;
t27 = t22.*(1.7e+1./1.0e+1);
t29 = t22.*(1.09e+2./1.0e+2);
t31 = atan(t30);
t32 = -t22.*(t6-xk1);
t34 = t15.*t20;
t36 = atan(t33);
t37 = t14.*t22;
t39 = t16.*t20;
t50 = t20.*(t6-xk1).*(-6.3e+1./8.0e+1);
t54 = t14.*t20.*(6.3e+1./8.0e+1);
t74 = t72.^2;
t79 = t78.^2;
t35 = atan(t32);
t38 = t15.*t23;
t40 = atan(t37);
t41 = t31.^2;
t42 = t16.*t23;
t43 = t34+1.0;
t46 = t39+1.0;
t47 = -t36;
t58 = t23.*(t6-xk1).*(6.3e+1./8.0e+1);
t59 = t14.*t23.*(6.3e+1./8.0e+1);
t60 = -t54;
t64 = t26+t50;
t81 = t4.*t31.*t78.*8.0e+3;
t85 = t4.*t31.*t78.*4.0e+4;
t44 = t35.^2;
t45 = t38+1.0;
t48 = t42+1.0;
t49 = -t40;
t51 = 1.0./t43;
t52 = delta+t47;
t56 = 1.0./t46;
t65 = t27+t58;
t66 = t28+t60;
t67 = t29+t59;
t80 = t4.*t35.*t76.*8.0e+3;
t83 = -t81;
t84 = t4.*t35.*t76.*4.0e+4;
t87 = atan(t85);
t99 = t5.*t41.*t79.*1.6e+9;
t55 = 1.0./t45;
t57 = delta+t49;
t61 = 1.0./t48;
t62 = t52.^2;
t82 = -t80;
t86 = atan(t84);
t88 = t4.*t52.*t73.*8.0e+3;
t91 = t4.*t52.*t73.*4.0e+4;
t95 = t87.*(6.0./5.0);
t98 = t5.*t44.*t77.*1.6e+9;
t101 = t99+1.0;
t112 = t4.*t19.*t56.*t73.*8.0e+3;
t113 = t4.*t19.*t51.*t78.*8.0e+3;
t116 = t4.*t51.*t64.*t78.*8.0e+3;
t118 = t4.*t56.*t66.*t73.*8.0e+3;
t63 = t57.^2;
t89 = t4.*t57.*t72.*8.0e+3;
t90 = -t88;
t93 = t4.*t57.*t72.*4.0e+4;
t94 = t86.*(6.0./5.0);
t96 = atan(t91);
t100 = t98+1.0;
t104 = t5.*t62.*t75.*1.6e+9;
t106 = 1.0./t101;
t114 = t4.*t22.*t55.*t76.*8.0e+3;
t115 = t4.*t22.*t61.*t72.*8.0e+3;
t117 = t4.*t55.*t65.*t76.*8.0e+3;
t119 = t4.*t61.*t67.*t72.*8.0e+3;
t121 = t83+t95;
t125 = (t81-t95).^2;
t92 = -t89;
t97 = atan(t93);
t102 = t96.*(6.0./5.0);
t105 = 1.0./t100;
t107 = t5.*t63.*t74.*1.6e+9;
t108 = t104+1.0;
t120 = t82+t94;
t123 = atan(t121);
t124 = (t80-t94).^2;
t127 = t125+1.0;
t148 = t4.*t19.*t51.*t78.*t106.*4.8e+4;
t156 = t4.*t51.*t64.*t78.*t106.*4.8e+4;
t103 = t97.*(6.0./5.0);
t109 = t107+1.0;
t110 = 1.0./t108;
t122 = atan(t120);
t126 = t124+1.0;
t129 = t123.*(1.1e+1./1.0e+1);
t131 = 1.0./t127;
t132 = t90+t102;
t137 = (t88-t102).^2;
t149 = t4.*t22.*t55.*t76.*t105.*4.8e+4;
t150 = -t148;
t157 = -t156;
t158 = t4.*t55.*t65.*t76.*t105.*4.8e+4;
t111 = 1.0./t109;
t128 = t122.*(1.1e+1./1.0e+1);
t130 = 1.0./t126;
t134 = cos(t129);
t135 = atan(t132);
t136 = t92+t103;
t139 = t137+1.0;
t140 = (t89-t103).^2;
t151 = -t149;
t152 = t4.*t19.*t56.*t73.*t110.*4.8e+4;
t159 = -t158;
t160 = t4.*t56.*t66.*t73.*t110.*4.8e+4;
t164 = t113+t150;
t168 = t116+t157;
t133 = cos(t128);
t138 = atan(t136);
t141 = t140+1.0;
t142 = t135.*(1.1e+1./1.0e+1);
t143 = 1.0./t139;
t153 = -t152;
t154 = t4.*t22.*t61.*t72.*t111.*4.8e+4;
t161 = -t160;
t162 = t4.*t61.*t67.*t72.*t111.*4.8e+4;
t166 = t114+t151;
t169 = t117+t159;
t144 = cos(t142);
t145 = t138.*(1.1e+1./1.0e+1);
t146 = 1.0./t141;
t155 = -t154;
t163 = -t162;
t165 = t112+t153;
t170 = t118+t161;
t147 = cos(t145);
t167 = t115+t155;
t171 = t119+t163;
t172 = mu.*t69.*t143.*t144.*t165.*(1.1e+1./1.0e+1);
t174 = mu.*t69.*t143.*t144.*t170.*(1.1e+1./1.0e+1);
t173 = mu.*t68.*t146.*t147.*t167.*(1.1e+1./1.0e+1);
t175 = mu.*t68.*t146.*t147.*t171.*(1.1e+1./1.0e+1);
t176 = t172+t173;
t177 = t174+t175;
mt1 = [(t2.*t176)./1.623e+3+mu.*t70.*t130.*t133.*t166.*6.777572396796057e-4+mu.*t71.*t131.*t134.*t164.*6.777572396796057e-4,t2.*t176.*5.275895450145208e-4-t3.*(t172-t173).*3.811713455953533e-4-mu.*t70.*t130.*t133.*t166.*9.051306873184898e-4-mu.*t71.*t131.*t134.*t164.*9.051306873184898e-4,-Vx+(t2.*t177)./1.623e+3-mu.*t70.*t130.*t133.*t169.*6.777572396796057e-4-mu.*t71.*t131.*t134.*t168.*6.777572396796057e-4];
mt2 = [t2.*t177.*5.275895450145208e-4-t3.*(t174-t175).*3.811713455953533e-4+mu.*t70.*t130.*t133.*t169.*9.051306873184898e-4+mu.*t71.*t131.*t134.*t168.*9.051306873184898e-4];
gradfx = reshape([mt1,mt2],2,2);
% end

% % -----------------------------------------------------------------

function gradfu = B_(delta)
%B_
%    GRADFU = B_(DELTA)

%    This function was generated by the Symbolic Math Toolbox version 24.2.
%    28-Jun-2025 15:18:15

gradfu = reshape([0.0,cos(delta).*4.956461056964821e-3,0.0,4.956461056964821e-3],[2,2]);
% end


% end
